simulink model "TanqueAguaBooleanoSimulacion"  (R2024b)
settings: Solver=VariableStepAuto  StartTime=0.0  StopTime=2000.0  RelTol=1e-3
settings Model: Creator=user  LastModifiedBy=user

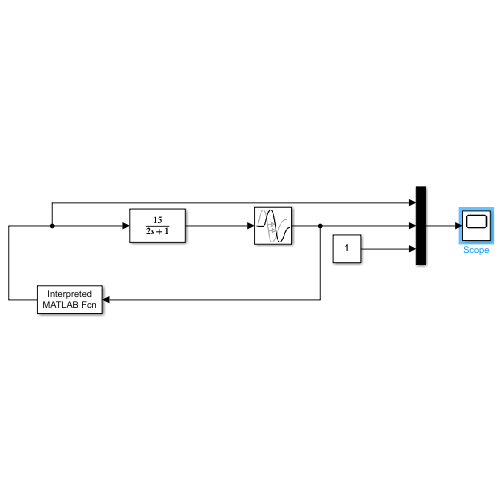
[thumbnail: Simulink's stored preview of the top-level diagram]
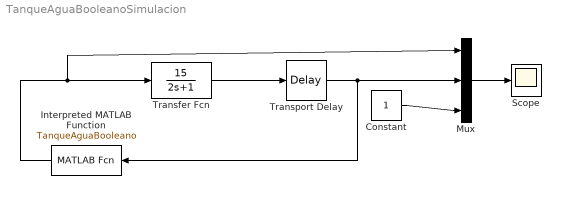
== system TanqueAguaBooleanoSimulacion ==
  Constant : Constant
  Interpreted MATLAB Function : MATLABFcn  MATLABFcn=TanqueAguaBooleano
  Mux : Mux  Inputs=3
  Scope : Scope
  Transfer Fcn : TransferFcn  Numerator=[15]  Denominator=[2 1]
  Transport Delay : TransportDelay  DelayTime=0.5
  wires:
  Constant/1 -> Mux/3
  Transfer Fcn/1 -> Transport Delay/1
  Transport Delay/1 -> Interpreted MATLAB Function/1, Mux/2
  Interpreted MATLAB Function/1 -> Mux/1, Transfer Fcn/1
  Mux/1 -> Scope/1
